simulink subsystem "Motor"  (R2023a)
settings: Solver=VariableStepAuto  StartTime=0.0  StopTime=10.0  RelTol=1e-3
values from neighbouring files (symbols this model uses):
  Km = 0.04025    [CoreXY_analysis_func.m]    (also in tuning.m)
undefined symbols (not defined in the file or in its folder): current_limit, L_terminal, R_terminal
libraries: cstblocks x1
settings Model: Creator=trent  LastModifiedBy=trent

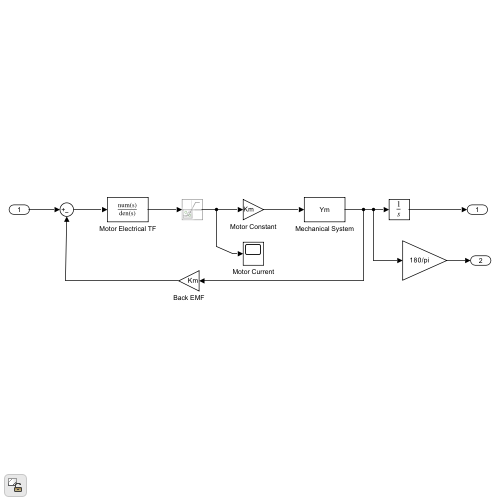
[thumbnail: Simulink's stored preview of the top-level diagram]
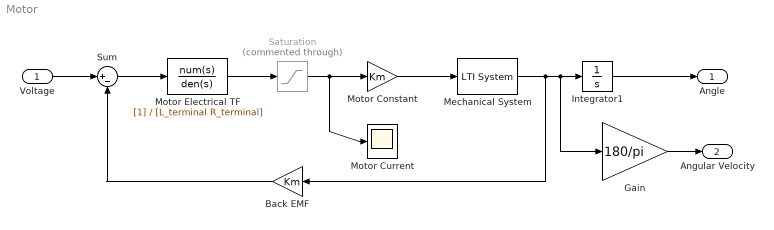
== system Motor ==
  Voltage : Inport
  Back EMF : Gain  Gain=Km
  Gain : Gain  Gain=180/pi
  Integrator1 : Integrator
  Mechanical System : cstblocks/LTI System  sys=Ym  IC=[]
  Motor Constant : Gain  Gain=Km
  Motor Current : Scope
  Motor Electrical TF : TransferFcn  Denominator=[L_terminal R_terminal]
  Saturation : Saturate  Commented=through  UpperLimit=current_limit  LowerLimit=-current_limit
  Sum : Sum  Inputs=|+-
  Angle : Outport
  Angular Velocity : Outport  Port=2
  wires:
  Motor Constant/1 -> Mechanical System/1
  Mechanical System/1 -> Back EMF/1, Gain/1, Integrator1/1
  Back EMF/1 -> Sum/2
  Saturation/1 -> Motor Constant/1, Motor Current/1
  Voltage/1 -> Sum/1
  Motor Electrical TF/1 -> Saturation/1
  Integrator1/1 -> Angle/1
  Sum/1 -> Motor Electrical TF/1
  Gain/1 -> Angular Velocity/1
